simulink model "pmmotor"  (R2023a)
settings: Solver=VariableStepAuto  StartTime=0.0  StopTime=10.0  RelTol=1e-3
libraries: spsIdealSwitchLib x8, spsDCVoltageSourceLib x2, spsStepperMotorLib x1, sps_lib x1
settings Model: Creator=acer  LastModifiedBy=acer

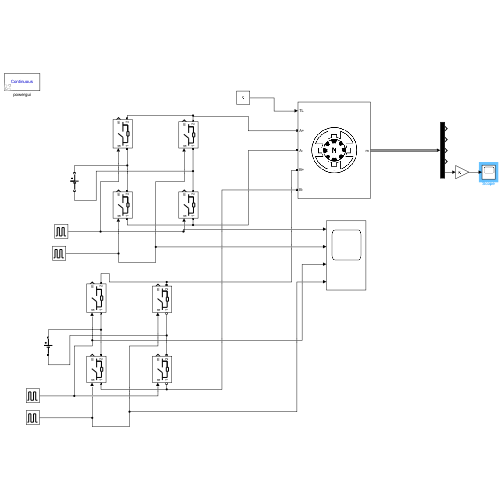
[thumbnail: Simulink's stored preview of the top-level diagram]
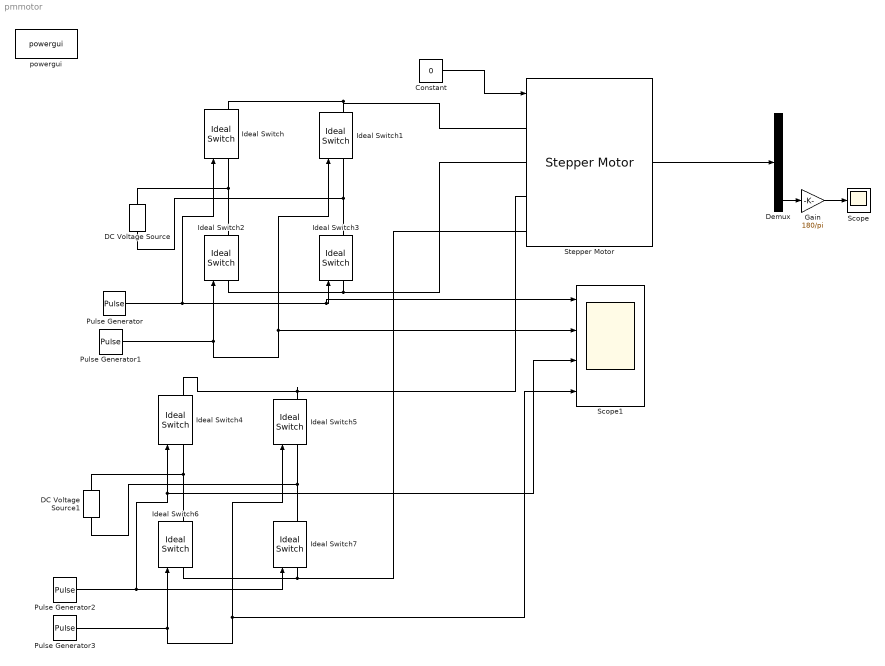
== system pmmotor ==
  Constant : Constant  Value=0
  DC Voltage Source : spsDCVoltageSourceLib/DC Voltage Source  Amplitude=25  Measurements=None
  DC Voltage Source1 : spsDCVoltageSourceLib/DC Voltage Source  Amplitude=25  Measurements=None
  Demux : Demux  Outputs=5
  Gain : Gain  Gain=180/pi
  Ideal Switch{,1..7} (8 alike) : spsIdealSwitchLib/Ideal Switch  Ron=0.001  Lon=0  IC=0  Rs=1e5  Cs=inf  Measurements=on
  Pulse Generator : DiscretePulseGenerator  PulseType=Time based  Period=8  PulseWidth=37.5  PhaseDelay=-1
  Pulse Generator1 : DiscretePulseGenerator  PulseType=Time based  Period=8  PulseWidth=37.5  PhaseDelay=3
  Pulse Generator2 : DiscretePulseGenerator  PulseType=Time based  Period=8  PulseWidth=37.5  PhaseDelay=1
  Pulse Generator3 : DiscretePulseGenerator  PulseType=Time based  Period=8  PulseWidth=37.5  PhaseDelay=5
  Scope : Scope
  Scope1 : Scope  NumInputPorts=4
  Stepper Motor : spsStepperMotorLib/Stepper Motor  MotorType=Permanent-magnet / Hybrid  NumberOfPhases_1=2  NumberOfPhases_2=3  PresetModel_1=<empty>  PresetModel_2=<empty>  L=10e-3  Lmax=10e-3  Lmin=2e-3  R=1.2  Step_angle=30  Psim=0.04  Tdm=0.02  J=1e-4/5  B=1e-3  w0=0  pos0=0  TsPowergui=0  TsBlock=-1
      settings: LibrarySourceBlock=sps_lib/Electrical Machines/Stepper Motor
  powergui : sps_lib/powergui  Priority=1  SimulationMode=Continuous  SampleTime=50e-6  frequency=60  Iterations=50  frequencyindice=0  Pbase=100e6  ErrMax=1e-4  UnitsV=kV  UnitsW=MW  buscounter=0  FunctionMessages=off  echomessages=off  EnableUseOfTLC=off  CurrentSourceSwitches=off  DisableSnubberDevices=off  DisableRonSwitches=off  DisableVfSwitches=off  DisplayEquations=off  AutomaticDiscreteSolvers=off  SolverType=Tustin/Backward Euler (TBE)  Interpol=off  ExternalGateDelay=off  methode=off  Ts=100  x0status=blocks  SPID=on  SwTol=0  HookPort=off  NonlinearTolerance=1e-4  nMaxIteration=100  ContinueOnMaxIteration=off  RestoreLinks=warning  ResistiveCurrentMeasurement=off  Frange=[0:2:500]  Ylog=off  Xlog=on  ShowGrid=off  save=off  variable=ZData  structure=0  ZoomFFT=off  StartTime=0.0  cycles=1  DisplayStyle=1  fundamental=60  FreqAxis=off  MaxFrequency=1000  frequencyindicesteady=1  RmsSteady=1  display=off
  wires:
  Stepper Motor/1 -> Demux/1
  Demux/5 -> Gain/1
  Constant/1 -> Stepper Motor/1
  Pulse Generator/1 -> Scope1/1, Ideal Switch3/1, Ideal Switch/1
  Pulse Generator1/1 -> Scope1/2, Ideal Switch1/1, Ideal Switch2/1
  Pulse Generator2/1 -> Ideal Switch7/1, Scope1/3, Ideal Switch4/1
  Pulse Generator3/1 -> Scope1/4, Ideal Switch5/1, Ideal Switch6/1
  Gain/1 -> Scope/1
  connections:
  Ideal Switch/LConn1 -- DC Voltage Source/RConn1 -- Ideal Switch2/RConn1
  Ideal Switch3/LConn1 -- Stepper Motor/LConn2 -- Ideal Switch2/LConn1
  Ideal Switch1/RConn1 -- Stepper Motor/LConn1 -- Ideal Switch/RConn1
  Ideal Switch1/LConn1 -- DC Voltage Source/LConn1 -- Ideal Switch3/RConn1
  Ideal Switch5/LConn1 -- DC Voltage Source1/LConn1 -- Ideal Switch7/RConn1
  Ideal Switch5/RConn1 -- Stepper Motor/LConn3 -- Ideal Switch4/RConn1
  Ideal Switch7/LConn1 -- Stepper Motor/LConn4 -- Ideal Switch6/LConn1
  Ideal Switch4/LConn1 -- DC Voltage Source1/RConn1 -- Ideal Switch6/RConn1
